simulink model "DirFeedthroughCal"  (R2025b)
settings: Solver=FixedStepDiscrete  StartTime=0.0  StopTime=Inf  FixedStep=0.01  RelTol=1e-3  EnableMultiTasking=on
undefined symbols (not defined in the file or in its folder): X, Y
libraries: MagLevTbx_BaseLib x11
settings Model: ExtModeTrigDuration=2  Creator=riccardo  LastModifiedBy=riccardo
settings SolverCC: AutoInsertRateTranBlk=on
settings OptimizationCC: EnhancedBackFolding=on  PassReuseOutputArgsAs=Individual arguments  ZeroExternalMemoryAtStartup=off  ZeroInternalMemoryAtStartup=off  MaxStackSize=64  OptimizeBlockOrder=speed  DifferentSizesBufferReuse=on  OptimizationCustomize=off  EfficientTunableParamExpr=on
settings DebuggingCC: ParameterTunabilityLossMsg=error
settings HardwareCC: ProdBitPerPointer=32.0  ProdBitPerSizeT=32.0  ProdBitPerPtrDiffT=32.0  ProdLargestAtomicInteger=Long  ProdLargestAtomicFloat=Double  ProdWordSize=32.0  ProdHWDeviceType=ARM Compatible->ARM Cortex
settings SFSimCC: MATLABDynamicMemAlloc=off
settings RTWCC: SystemTargetFile=ert.tlc  HardwareBoard=Teensy 4.1 (Arduino Compatible)  TemplateMakefile=ert_default_tmf  Toolchain=Arduino ARM M7  BuildConfiguration=Faster Runs  Description=Embedded Coder
settings CodeAppCC: ForceParamTrailComments=on  IgnoreCustomStorageClasses=off  OperatorAnnotations=on  SimulinkDataObjDesc=on  SFDataObjDesc=on  InsertBlockDesc=on
settings ERTTargetCC: ExtModeTransport=3.0  ExtModeStaticAlloc=on  ExtModeAutomaticAllocSize=off  ExtModeStaticAllocSize=65536.0  ExtModeMexFile=ext_xcp  ExtModeIntrfLevel=Level2 - Open  InlinedParameterPlacement=Hierarchical  RootIOFormat=Structure reference  TargetLangStandard=C99 (ISO)  SupportContinuousTime=on  SupportVariableSizeSignals=on

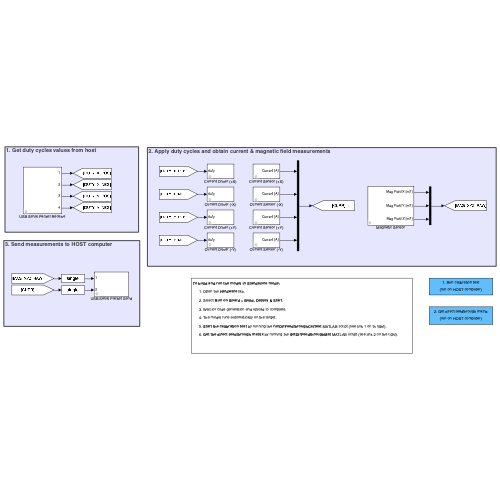
[thumbnail: Simulink's stored preview of the top-level diagram]
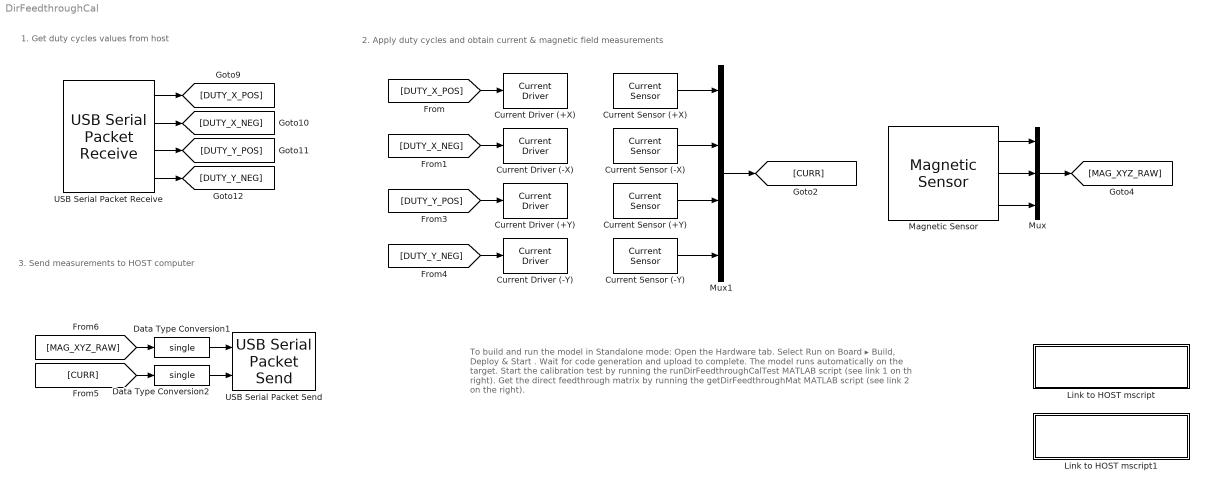
== system DirFeedthroughCal ==
  note: 3. Send measurements to HOST computer
  note: 1. Get duty cycles values from host
  note: 2. Apply duty cycles and obtain current & magnetic field measurements
  note: To build and run the model in Standalone mode:
      | Open the Hardware tab.
      | Select Run on Board ▸ Build, Deploy & Start .
      | Wait for code generation and upload to complete.
      | The model runs automatically on the target.
      | Start the calibration test by running the runDirFeedthroughCalTest MATLAB script (see link 1 on th right).
      | Get the direct feedthrough matrix by running the getDirFeedthroughMat MATLAB script (see link 2 on the right).
  Current Driver (+X) : MagLevTbx_BaseLib/Outputs/Current Driver  driverId=+X  sampleTime=-1  showEnablePort=off
      settings: SourceProductName=MagLev Toolbox
  Current Driver (+Y) : MagLevTbx_BaseLib/Outputs/Current Driver  driverId=+Y  sampleTime=-1  showEnablePort=off
      settings: SourceProductName=MagLev Toolbox
  Current Driver (-X) : MagLevTbx_BaseLib/Outputs/Current Driver  driverId=-X  sampleTime=-1  showEnablePort=off
      settings: SourceProductName=MagLev Toolbox
  Current Driver (-Y) : MagLevTbx_BaseLib/Outputs/Current Driver  driverId=-Y  sampleTime=-1  showEnablePort=off
      settings: SourceProductName=MagLev Toolbox
  Current Sensor (+X) : MagLevTbx_BaseLib/Inputs/Current Sensor  sensorId=+X  sampleTime=-1  showEnablePort=off
      settings: SourceProductName=MagLev Toolbox
  Current Sensor (+Y) : MagLevTbx_BaseLib/Inputs/Current Sensor  sensorId=+Y  sampleTime=-1  showEnablePort=off
      settings: SourceProductName=MagLev Toolbox
  Current Sensor (-X) : MagLevTbx_BaseLib/Inputs/Current Sensor  sensorId=-X  sampleTime=-1  showEnablePort=off
      settings: SourceProductName=MagLev Toolbox
  Current Sensor (-Y) : MagLevTbx_BaseLib/Inputs/Current Sensor  sensorId=-Y  sampleTime=-1  showEnablePort=off
      settings: SourceProductName=MagLev Toolbox
  Data Type Conversion1 : DataTypeConversion  OutDataTypeStr=single  SaturateOnIntegerOverflow=off  RndMeth=Floor
  Data Type Conversion2 : DataTypeConversion  OutDataTypeStr=single  SaturateOnIntegerOverflow=off  RndMeth=Floor
  Link to HOST mscript : Subsystem
      settings: OpenFcn=|
      | %  get toolbox base dir
      | info = MagLevTbx_Info();
      | 
      | %  path to HOST matlab script
      | mscriptpath = fullfile( ...
      | info.rootDir, ...
      | 'Examples', ...
      | 'Ctrl_Test', ...
      | 'Standalone', ...
      | 'runDirFeedthroughCalTest'  );
      | 
      | %  open script
      | edit( mscriptpath );
      | 
      | %  clear temp vars
      | clear info mscriptpath;
      mask Display:
      | disp(['1. Run calibration test\n\n' ...
      |     '(run on HOST computer)'])
  Link to HOST mscript1 : Subsystem
      settings: OpenFcn=|
      | %  get toolbox base dir
      | info = MagLevTbx_Info();
      | 
      | %  path to HOST matlab script
      | mscriptpath = fullfile( ...
      | info.rootDir, ...
      | 'Examples', ...
      | 'Ctrl_Test', ...
      | 'Standalone', ...
      | 'getDirFeedthroughMat'  );
      | 
      | %  open script
      | edit( mscriptpath );
      | 
      | %  clear temp vars
      | clear info mscriptpath;
      mask Display:
      | disp(['2. Get direct feedthrough matrix\n\n' ...
      |     '(run on HOST computer)'])
  Magnetic Sensor : MagLevTbx_BaseLib/Inputs/Magnetic Sensor  sensorId=Sensor 7  sampleTime=-1  showEnablePort=off
      settings: SourceProductName=MagLev Toolbox
  Mux : Mux  Inputs=3
  Mux1 : Mux
  USB Serial Packet Receive : MagLevTbx_BaseLib/Communication/USB Serial Packet Receive  outputMode=HOLD Outputs  showStatusPort=off  packetSpec={'int16', 'int16', 'int16', 'int16'}  cobsEncoded=on  nullTerminated=on  sampleTime=-1  showEnablePort=off
      settings: SourceProductName=MagLev Toolbox
  USB Serial Packet Send : MagLevTbx_BaseLib/Communication/USB Serial Packet Send  waitDTR=on  packetSpec={'3*single', '4*single'}  cobsEncoded=on  nullTerminated=on  sampleTime=-1  showEnablePort=off
      settings: SourceProductName=MagLev Toolbox
  wires:
  Data Type Conversion1/1 -> USB Serial Packet Send/1
  Data Type Conversion2/1 -> USB Serial Packet Send/2
  Magnetic Sensor/1 -> Mux/1
  Magnetic Sensor/2 -> Mux/2
  Magnetic Sensor/3 -> Mux/3
  Current Sensor (+X)/1 -> Mux1/1
  Current Sensor (-X)/1 -> Mux1/2
  Current Sensor (+Y)/1 -> Mux1/3
  Current Sensor (-Y)/1 -> Mux1/4
  [DUTY_X_POS] -> Current Driver (+X)/1
  [DUTY_X_NEG] -> Current Driver (-X)/1
  [DUTY_Y_POS] -> Current Driver (+Y)/1
  [DUTY_Y_NEG] -> Current Driver (-Y)/1
  USB Serial Packet Receive/1 -> [DUTY_X_POS]
  USB Serial Packet Receive/2 -> [DUTY_X_NEG]
  USB Serial Packet Receive/3 -> [DUTY_Y_POS]
  USB Serial Packet Receive/4 -> [DUTY_Y_NEG]
  Mux/1 -> [MAG_XYZ_RAW]
  Mux1/1 -> [CURR]
  [CURR] -> Data Type Conversion2/1
  [MAG_XYZ_RAW] -> Data Type Conversion1/1

== system DirFeedthroughCal/Link to HOST mscript ==

== system DirFeedthroughCal/Link to HOST mscript1 ==
